simulink model "mpcVDAutoParkingRRT"  (R2023a)
settings: Solver=VariableStepAuto  StartTime=0.0  StopTime=Duration  RelTol=1e-3
values from neighbouring files (symbols this model uses):
  distToCenter = 0.5*egoWheelbase    [ParallelParkingUsingRRTPlannerAndMPCTrackingController1.m]
  Duration = 14    [ParallelParkingUsingRRTPlannerAndMPCTrackingController1.m]
  egoInitialPose = [7,3.1,0]    [ParallelParkingUsingRRTPlannerAndMPCTrackingController1.m]
  pTracking = 10    [ParallelParkingUsingRRTPlannerAndMPCTrackingController1.m]
  Ts = 0.1    [ParallelParkingUsingRRTPlannerAndMPCTrackingController1.m]
  Xref = [xRef(2:p+1,:);repmat(xRef(end,:),Tsteps-p,1)]    [ParallelParkingUsingRRTPlannerAndMPCTrackingController1.m]
libraries: autolibshared x1, mpclib x1, simulink_extras x1
settings Model: Creator=The MathWorks, Inc.  LastModifiedBy=The MathWorks, Inc.
settings SolverCC: AlgebraicLoopSolver=TrustRegion
settings DebuggingCC: UnconnectedInputMsg=warning  UnconnectedOutputMsg=warning  UnconnectedLineMsg=warning
settings ModelReferenceCC: EnableRefExpFcnMdlSchedulingChecks=on

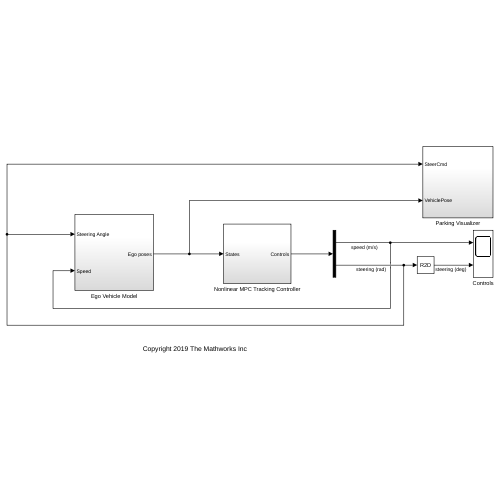
[thumbnail: Simulink's stored preview of the top-level diagram]
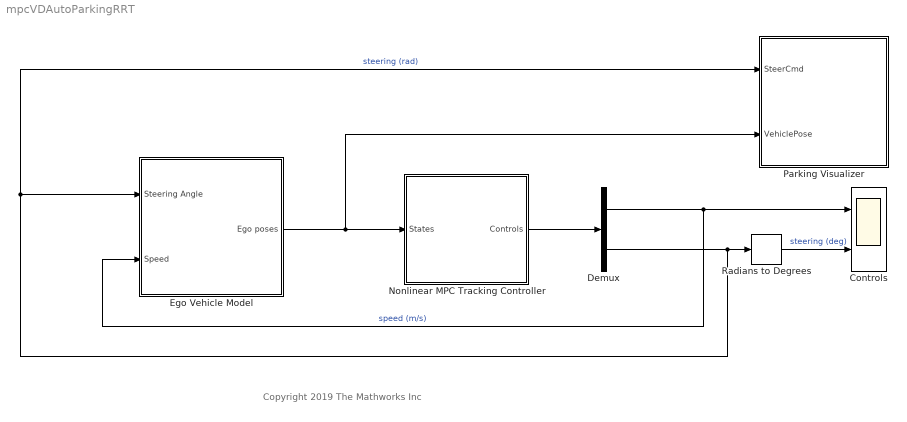
== system mpcVDAutoParkingRRT ==
  note: Copyright 2019 The Mathworks Inc
  Controls : Scope  NumInputPorts=2
  Demux : Demux  Outputs=[1 1]
  Ego Vehicle Model : Subsystem
  Nonlinear MPC Tracking Controller : Subsystem
  Parking Visualizer : Subsystem
  Radians to Degrees : simulink_extras/Transformations/Radians to Degrees
  wires:
  Radians to Degrees/1 -> Controls/2  "steering (deg)"
  Demux/2 -> Parking Visualizer/1(SteerCmd), Ego Vehicle Model/1(Steering Angle), Radians to Degrees/1  "steering (rad)"
  Demux/1 -> Ego Vehicle Model/2(Speed), Controls/1  "speed (m/s)"
  Ego Vehicle Model/1(Ego poses) -> Parking Visualizer/2(VehiclePose), Nonlinear MPC Tracking Controller/1(States)
  Nonlinear MPC Tracking Controller/1(Controls) -> Demux/1

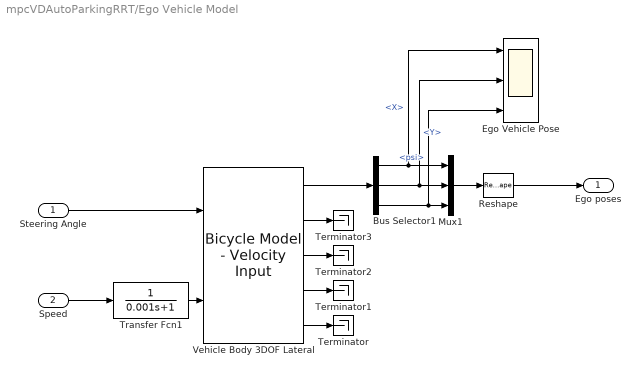
== system mpcVDAutoParkingRRT/Ego Vehicle Model ==
  Steering Angle : Inport
  Speed : Inport  Port=2
  Bus Selector1 : BusSelector  OutputSignals=InertFrm.RearAxl.Disp.X,InertFrm.RearAxl.Disp.Y,InertFrm.Cg.Ang.psi
  Ego Vehicle Pose : Scope  NumInputPorts=3
  Mux1 : Mux  Inputs=3
  Reshape : Reshape  OutputDimensionality=Customize  OutputDimensions=[3,1]
  Terminator{,1..3} (4 alike) : Terminator
  Transfer Fcn1 : TransferFcn  Numerator=1  Denominator=[0.001 1]
  Vehicle Body 3DOF Lateral : autolibshared/Bicycle Model - Velocity Input  trackMode=Single (bicycle)  inputMode=External longitudinal forces  frontSteerMode=on  rearSteerMode=off  windMode=off  muMode=off  extFMode=off  extMMode=off  aMode=3  NF=2  NR=2  m=2000  a=1.4  b=1.4  h=0.35  X_o=egoInitialPose(1)+distToCenter*cos(egoInitialPose(3))  xdot_o=0  CalphaMode=off  sigmaMode=on  w=[1.4,1.4]  Cy_f=12e3  Cy_r=11e3  sigma_f=.1  sigma_r=.1  alpha_f_brk=[-.1 .1]  Cy_f_data=[-9e3 9e3]  alpha_r_brk=[-.1 .1]  Cy_r_data=[-9e3 9e3]  Y_o=egoInitialPose(2)+distToCenter*sin(egoInitialPose(3))  ydot_o=0  Izz=4000  psi_o=egoInitialPose(3)  r_o=0  Af=0  Cd=.3  Cl=.1  Cpm=.1  beta_w=[0:0.01:0.3]  Cs=[0:0.03:0.9]  Cym=[0:0.01:0.3]  Pabs=101325  Tair=273  g=9.81  mu=1  xdot_tol=0.01  Fznom=5000  Fxtire_sat=1e6  Fytire_sat=1e6  longOff=0  latOff=0  vertOff=0
  Ego poses : Outport
  wires:
  Mux1/1 -> Reshape/1
  Vehicle Body 3DOF Lateral/2 -> Terminator3/1
  Bus Selector1/1 -> Ego Vehicle Pose/1, Mux1/1  "<X>"
  Vehicle Body 3DOF Lateral/5 -> Terminator/1
  Vehicle Body 3DOF Lateral/1 -> Bus Selector1/1
  Vehicle Body 3DOF Lateral/3 -> Terminator2/1
  Bus Selector1/2 -> Ego Vehicle Pose/2, Mux1/2  "<Y>"
  Vehicle Body 3DOF Lateral/4 -> Terminator1/1
  Bus Selector1/3 -> Ego Vehicle Pose/3, Mux1/3  "<psi>"
  Transfer Fcn1/1 -> Vehicle Body 3DOF Lateral/2
  Reshape/1 -> Ego poses/1
  Steering Angle/1 -> Vehicle Body 3DOF Lateral/1
  Speed/1 -> Transfer Fcn1/1

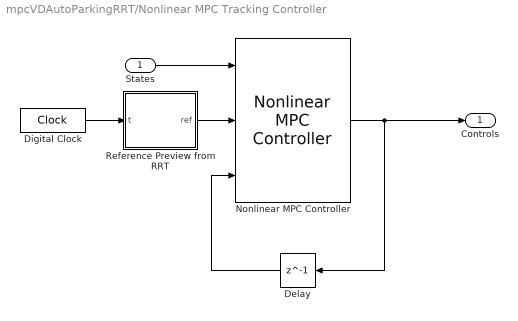
== system mpcVDAutoParkingRRT/Nonlinear MPC Tracking Controller ==
  States : Inport
  Delay : Delay  DelayLength=1
  Digital Clock : DigitalClock  SampleTime=Ts
  Nonlinear MPC Controller : mpclib/Nonlinear MPC Controller  SCDEnableBlockLinearizationSpecification=on  nlmpcobj=nlobjTracking  UseObjectTs=on  UseMEX=on  mexname='parkingRRTMex'  md_enabled=off  mvtarget_enabled=off  param_enabled=off  cost_enabled=off  mvseq_enabled=off  stateseq_enabled=off  ovseq_enabled=off  slack_enabled=off  status_enabled=off  ov_min=off  ov_max=off  mv_min=off  mv_max=off  mvrate_min=off  mvrate_max=off  state_min=off  state_max=off  ov_weight=off  mv_weight=off  mvrate_weight=off  ecr_weight=off  nlp_initialize=off
  Reference Preview from RRT : MATLAB Function  TreatAsAtomicUnit=on
  Controls : Outport
  wires:
  Reference Preview from RRT/1(ref) -> Nonlinear MPC Controller/2
  Nonlinear MPC Controller/1 -> Delay/1, Controls/1
  Delay/1 -> Nonlinear MPC Controller/3
  States/1 -> Nonlinear MPC Controller/1
  Digital Clock/1 -> Reference Preview from RRT/1(t)

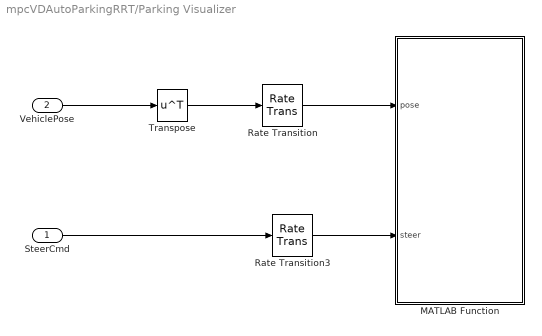
== system mpcVDAutoParkingRRT/Parking Visualizer ==
  SteerCmd : Inport
  VehiclePose : Inport  Port=2
  MATLAB Function : MATLAB Function  TreatAsAtomicUnit=on
  Rate Transition : RateTransition  OutPortSampleTime=Tv
  Rate Transition3 : RateTransition  OutPortSampleTime=Tv
  Transpose : Math  Operator=transpose
  wires:
  Rate Transition/1 -> MATLAB Function/1(pose)
  VehiclePose/1 -> Transpose/1
  Rate Transition3/1 -> MATLAB Function/2(steer)
  SteerCmd/1 -> Rate Transition3/1
  Transpose/1 -> Rate Transition/1

== matlab function mpcVDAutoParkingRRT/Nonlinear MPC Tracking Controller/Reference Preview from RRT ==
  data: t input; ref output; Ts parameter; Duration parameter; pTracking parameter; Xref parameter
function ref = fcn(t,Ts,Duration,pTracking,Xref)
Tend = Duration;
T = t+(1:pTracking)*Ts;
T = min(T,Tend);
time = Ts*(1:length(Xref));
ref = interp1(time,Xref,T);

== matlab function mpcVDAutoParkingRRT/Parking Visualizer/MATLAB Function ==
  data: pose input; steer input
function visualizeParking(pose, steer)

%visualizePath Display simulation results.

coder.extrinsic('helperSLVisualizeParking');

helperSLVisualizeParking(pose, steer);
